simulink model "MotionBlockWithExternalComponents"  (R2023b)
settings: Solver=ode45  StartTime=0.0  StopTime=100.0  RelTol=1e-3
values from neighbouring files (symbols this model uses):
  Cnb0 = C3 * C2 * C1    [InitializeModel.m]
  Fx = 600    [InitializeModel.m]
  Fy = 10000    [InitializeModel.m]
  Fz = -9.81    [InitializeModel.m]
  Jxx = J(1,1)    [InitializeModel.m]
  Jxz = J(1,3)    [InitializeModel.m]
  Jyy = J(2,2)    [InitializeModel.m]
  Jzz = J(3,3)    [InitializeModel.m]
  LL = 1000    [InitializeModel.m]
  MM = 10    [InitializeModel.m]
  NN = 1000    [InitializeModel.m]
  q0 = angle2quat(yaw,pitch,roll)    [InitializeModel.m]
  x0 = [6378100;0;0]    [InitializeModel.m]
libraries: matrix_library x1
settings Model: SnapshotBufferSize=5  SnapshotInterval=5  Creator=prafulsigdel  LastModifiedBy=prafulsigdel

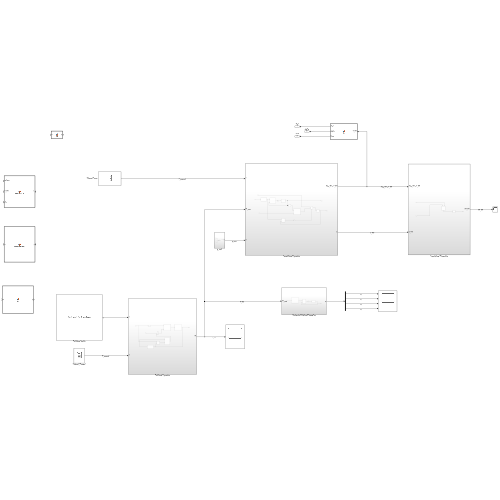
[thumbnail: Simulink's stored preview of the top-level diagram]
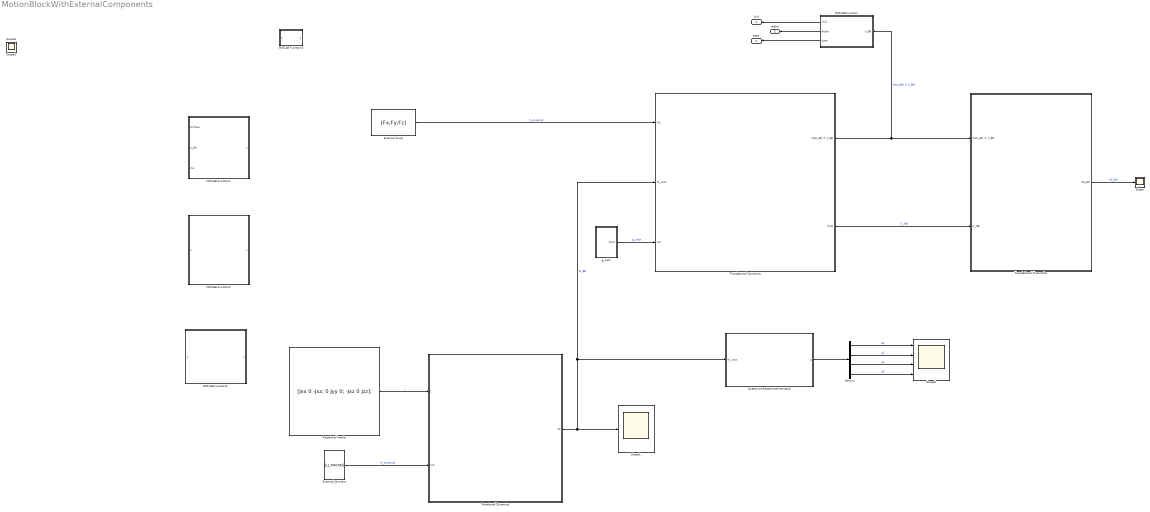
== system MotionBlockWithExternalComponents ==
  Demux : Demux
  External Force : Constant  Value=[Fx;Fy;Fz]  VectorParams1D=off
  External_Moment : Constant  Value=[LL;MM;NN]  VectorParams1D=off
  MATLAB Function : MATLAB Function  TreatAsAtomicUnit=on
  MATLAB Function1 : MATLAB Function  TreatAsAtomicUnit=on
  MATLAB Function2 : MATLAB Function  TreatAsAtomicUnit=on
  MATLAB Function3 : MATLAB Function  TreatAsAtomicUnit=on
  MATLAB Function4 : MATLAB Function  TreatAsAtomicUnit=on
  QuaternionRotationalKinematics : Subsystem
  Rotational Dynamics : Subsystem
  Rotational Inertia : Constant  Value=[Jxx 0 -Jxz; 0 Jyy 0; -Jxz 0 Jzz];  VectorParams1D=off
  Scope{,1,3..4} (4 alike) : Scope
  Scope2 : Scope  NumInputPorts=4
  Translational Dynamics : Subsystem
  Translational Kinematics : Subsystem
  g_vect : Subsystem
  Vinf : Outport
  alpha : Outport  Port=2
  beta : Outport  Port=3
  wires:
  External_Moment/1 -> Rotational Dynamics/2(In2)  "M_external"
  Rotational Dynamics/1(W) -> QuaternionRotationalKinematics/1(W_vect), Translational Dynamics/2(W_vect), Scope1/1  "W_BE"
  Demux/1 -> Scope2/1  "q0"
  QuaternionRotationalKinematics/1(q) -> Demux/1
  Demux/2 -> Scope2/2  "q1"
  Demux/4 -> Scope2/4  "q3"
  Demux/3 -> Scope2/3  "q2"
  External Force/1 -> Translational Dynamics/1(In1)  "F_external"
  g_vect/1(Out1) -> Translational Dynamics/3(In3)  "g_vect"
  Translational Kinematics/1(XN_BN) -> Scope/1  "XN_BN"
  Translational Dynamics/1(Xdot_BN = V_BN) -> MATLAB Function/1(V_BN), Translational Kinematics/1(Xdot_BN = V_BN)  "Xdot_BN = V_BN"
  Translational Dynamics/2(Out1) -> Translational Kinematics/2(C_NB)  "C_NB"
  Rotational Inertia/1 -> Rotational Dynamics/1(J)  "J"
  MATLAB Function/1(Vinf) -> Vinf/1
  MATLAB Function/2(alpha) -> alpha/1
  MATLAB Function/3(beta) -> beta/1

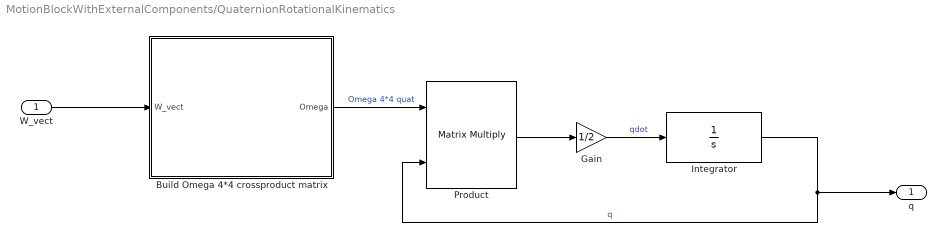
== system MotionBlockWithExternalComponents/QuaternionRotationalKinematics ==
  W_vect : Inport
  "Build Omega 4*4 crossproduct matrix " : MATLAB Function  TreatAsAtomicUnit=on
  Gain : Gain  Gain=1/2
  Integrator : Integrator  InitialCondition=q0
  Product : Product  Multiplication=Matrix(*)
  q : Outport
  wires:
  Gain/1 -> Integrator/1  "qdot"
  Product/1 -> Gain/1
  W_vect/1 -> "Build Omega 4*4 crossproduct matrix "/1(W_vect)
  Integrator/1 -> q/1, Product/2  "q"
  "Build Omega 4*4 crossproduct matrix "/1(Omega) -> Product/1  "Omega 4*4 quat"

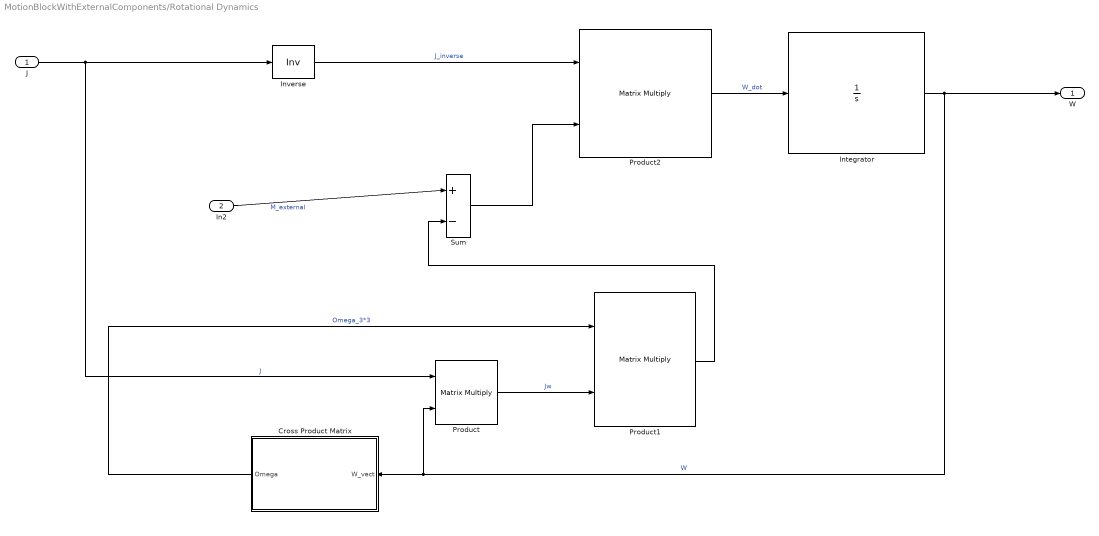
== system MotionBlockWithExternalComponents/Rotational Dynamics ==
  J : Inport
  In2 : Inport  Port=2
  Cross Product Matrix : MATLAB Function  TreatAsAtomicUnit=on
  Integrator : Integrator  InitialCondition=[10;0;0]  ZeroCross=off
  Inverse : Product  Inputs=/  Multiplication=Matrix(*)
  Product : Product  Multiplication=Matrix(*)
  Product1 : Product  Multiplication=Matrix(*)
  Product2 : Product  Multiplication=Matrix(*)
  Sum : Sum  Inputs=|+-
  W : Outport
  wires:
  Sum/1 -> Product2/2
  Inverse/1 -> Product2/1  "J_inverse"
  Product/1 -> Product1/2  "Jw"
  Cross Product Matrix/1(Omega) -> Product1/1  "Omega_3*3"
  Product2/1 -> Integrator/1  "W_dot"
  Product1/1 -> Sum/2
  Integrator/1 -> W/1, Product/2, Cross Product Matrix/1(W_vect)  "W"
  In2/1 -> Sum/1  "M_external"
  J/1 -> Inverse/1, Product/1  "J"

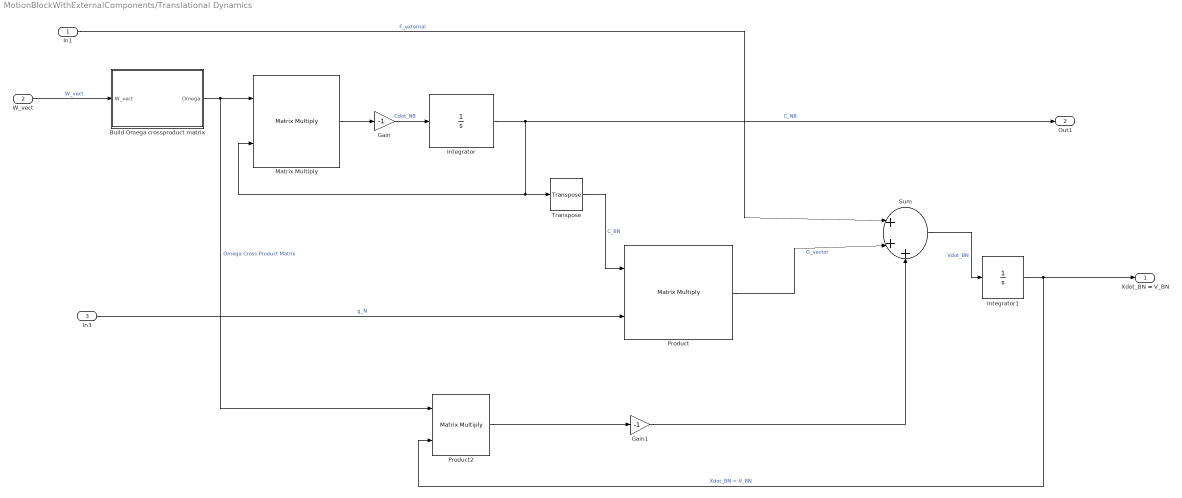
== system MotionBlockWithExternalComponents/Translational Dynamics ==
  In1 : Inport
  W_vect : Inport  Port=2
  In3 : Inport  Port=3
  "Build Omega crossproduct matrix " : MATLAB Function  TreatAsAtomicUnit=on
  Gain : Gain  Gain=-1
  Gain1 : Gain  Gain=-1
  Integrator : Integrator  InitialCondition=Cnb0
  Integrator1 : Integrator  InitialCondition=[100;0;0]
  Matrix Multiply : Product  Multiplication=Matrix(*)
  Product : Product  Multiplication=Matrix(*)
  Product2 : Product  Multiplication=Matrix(*)
  Sum : Sum  Inputs=|+++
  Transpose : matrix_library/Transpose
  Xdot_BN = V_BN : Outport
  Out1 : Outport  Port=2
  wires:
  In3/1 -> Product/2  "g_N"
  Sum/1 -> Integrator1/1  "Vdot_BN"
  Transpose/1 -> Product/1  "C_BN"
  Gain1/1 -> Sum/3
  Product/1 -> Sum/2  "G_vector"
  Matrix Multiply/1 -> Gain/1
  W_vect/1 -> "Build Omega crossproduct matrix "/1(W_vect)  "W_vect"
  In1/1 -> Sum/1  "F_external"
  Integrator/1 -> Out1/1, Matrix Multiply/2, Transpose/1  "C_NB"
  Gain/1 -> Integrator/1  "Cdot_NB"
  "Build Omega crossproduct matrix "/1(Omega) -> Matrix Multiply/1, Product2/1  "Omega Cross Product Matrix"
  Integrator1/1 -> Xdot_BN = V_BN/1, Product2/2  "Xdot_BN = V_BN"
  Product2/1 -> Gain1/1

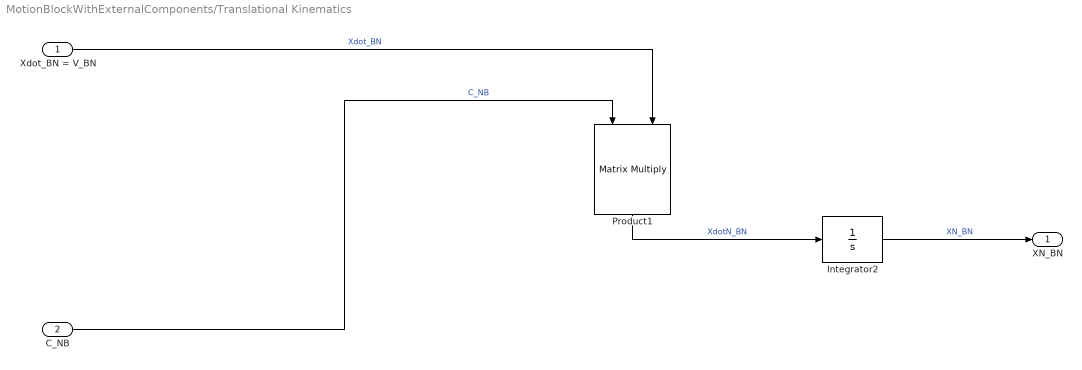
== system MotionBlockWithExternalComponents/Translational Kinematics ==
  Xdot_BN = V_BN : Inport
  C_NB : Inport  Port=2
  Integrator2 : Integrator  InitialCondition=x0
  Product1 : Product  Multiplication=Matrix(*)
  XN_BN : Outport
  wires:
  C_NB/1 -> Product1/1  "C_NB"
  Integrator2/1 -> XN_BN/1  "XN_BN"
  Xdot_BN = V_BN/1 -> Product1/2  "Xdot_BN"
  Product1/1 -> Integrator2/1  "XdotN_BN"

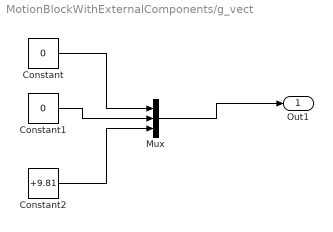
== system MotionBlockWithExternalComponents/g_vect ==
  Constant : Constant  Value=0
  Constant1 : Constant  Value=0
  Constant2 : Constant  Value=+9.81
  Mux : Mux  Inputs=3
  Out1 : Outport
  wires:
  Constant2/1 -> Mux/3
  Constant/1 -> Mux/1
  Constant1/1 -> Mux/2
  Mux/1 -> Out1/1

== matlab function MotionBlockWithExternalComponents/Rotational Dynamics/Cross Product Matrix ==
  data: W_vect input; Omega output
function Omega = fcn(W_vect)

p = W_vect(1);
q = W_vect(2);
r = W_vect(3);


Omega = [0 -r q;
    r 0 -p;
    -q p 0];

== matlab function MotionBlockWithExternalComponents/Translational Dynamics/Build Omega crossproduct matrix  ==
  data: W_vect input; Omega output
function Omega = fcn(W_vect)

p = W_vect(1);
q = W_vect(2);
r = W_vect(3);


Omega = [0 -r q;
    r 0 -p;
    -q p 0];

== matlab function MotionBlockWithExternalComponents/QuaternionRotationalKinematics/Build Omega 4*4 crossproduct matrix  ==
  data: W_vect input; Omega output
function Omega = fcn(W_vect)

wx = W_vect(1);
wy = W_vect(2);
wz = W_vect(3);


Omega = [0 -wx -wy -wz;
    wx 0 wz -wy;
    wy -wz 0 wx;
    wz wy -wx 0];

== matlab function MotionBlockWithExternalComponents/MATLAB Function ==
  data: V_BN input; Vinf output; alpha output; beta output
function [Vinf,alpha,beta]= fcn(V_BN)

alpha = atan2(V_BN(3),V_BN(1));
u = norm(V_BN);
X = V_BN(2)/u;
beta = asin(X);
Vinf = u;

== matlab function MotionBlockWithExternalComponents/MATLAB Function1 ==
  data: surface input; V_BN input; L output; rho input
function L = calculate_lift(surface,V_BN,rho)
Cls = surface.CL0 + surface.CLa * (surface.i-asin());

L = Cls * 0.5 * rho * norm(V_BN)^2 * surface.area;

== matlab function MotionBlockWithExternalComponents/MATLAB Function2 ==
  data: u input; y output
function y = calculate_drag(u)

y = u;

== matlab function MotionBlockWithExternalComponents/MATLAB Function3 ==
  data: u input; y output
function y = fcn(u)

y = u;

== matlab function MotionBlockWithExternalComponents/MATLAB Function4 ==
  data: u input; y output
function y = fcn(u)

y = u;
